simulink model "core1_simulator"  (R2024b)
settings: Solver=FixedStepDiscrete  StartTime=0.0  StopTime=50  FixedStep=0.001  RelTol=1e-3
undefined symbols (not defined in the file): DiscIntNeverNeededParam, task_table_data
settings Model: Creator=bianca  LastModifiedBy=bianca
settings OptimizationCC: BlockReduction=off

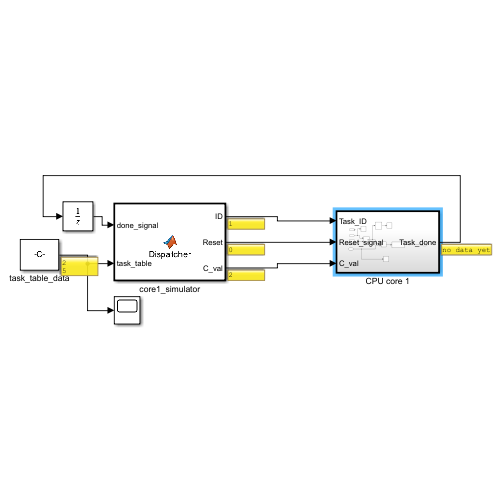
[thumbnail: Simulink's stored preview of the top-level diagram]
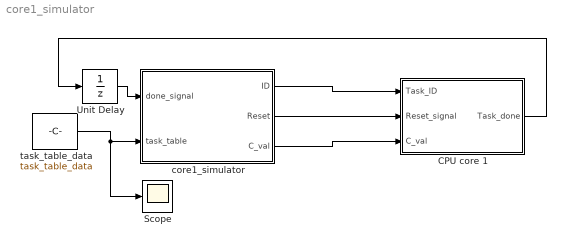
== system core1_simulator ==
  CPU core 1 : Subsystem  TreatAsAtomicUnit=on
  Scope : Scope
  Unit Delay : UnitDelay  SampleTime=0.001  HasFrameUpgradeWarning=on
  core1_simulator : MATLAB Function  TreatAsAtomicUnit=on
  task_table_data : Constant  Value=task_table_data  VectorParams1D=off  OutDataTypeStr=double  SampleTime=50
  wires:
  core1_simulator/1(ID) -> CPU core 1/1(Task_ID)
  core1_simulator/2(Reset) -> CPU core 1/2(Reset_signal)
  CPU core 1/1(Task_done) -> Unit Delay/1
  task_table_data/1 -> Scope/1, core1_simulator/2(task_table)
  Unit Delay/1 -> core1_simulator/1(done_signal)
  core1_simulator/3(C_val) -> CPU core 1/3(C_val)

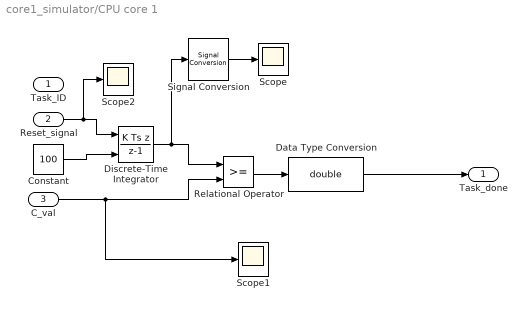
== system core1_simulator/CPU core 1 ==
  Task_ID : Inport
  Reset_signal : Inport  Port=2  PortDimensions=1
  C_val : Inport  Port=3  SampleTime=0.001
  Constant : Constant  Value=100  VectorParams1D=off  SampleTime=0.001
  Data Type Conversion : DataTypeConversion  OutDataTypeStr=double  SaturateOnIntegerOverflow=off  RndMeth=Floor
  Discrete-Time Integrator : DiscreteIntegrator  IntegratorMethod=Integration: Backward Euler  ExternalReset=rising  InitialCondition=0.001  SampleTime=0.001  ICPrevOutput=DiscIntNeverNeededParam  ICPrevScaledInput=DiscIntNeverNeededParam
  Relational Operator : RelationalOperator  OutDataTypeStr=boolean  RndMeth=Simplest  InputSameDT=off
  Scope : Scope
  Scope1 : Scope
  Scope2 : Scope
  Signal Conversion : SignalConversion  OverrideOpt=off
  Task_done : Outport
  wires:
  Reset_signal/1 -> Scope2/1, Discrete-Time Integrator/1
  Discrete-Time Integrator/1 -> Signal Conversion/1, Relational Operator/1
  Relational Operator/1 -> Data Type Conversion/1
  Data Type Conversion/1 -> Task_done/1
  Constant/1 -> Discrete-Time Integrator/2
  C_val/1 -> Relational Operator/2, Scope1/1
  Signal Conversion/1 -> Scope/1

== matlab function core1_simulator/core1_simulator ==
  data: done_signal input size=1; ID output; task_table input; Reset output size=1; C_val output size=1
function [ID, Reset, C_val] = Dispatcher(done_signal, task_table)

    ID = 1.0;
    C_val = 0.0;
    Reset = 0.0;

    persistent current_idx;
    persistent last_done_state;

    if isempty(current_idx)
        current_idx = 1;
        last_done_state = 0;
    end

    current_done = double(any(done_signal > 0.5));

    if isempty(last_done_state)
        Reset = 0.0;
    elseif (current_done == 1) && (last_done_state == 0)
        current_idx = current_idx + 1;
        Reset = 1.0;
    else
        Reset = 0.0;
    end
    
    % task is done, move to the next one
    if (current_done == 1) && (last_done_state == 0)
        current_idx = current_idx + 1;
        Reset = 1.0;
    else
        Reset = 0.0;
    end
   
    num_tasks = size(task_table, 1);

    if current_idx > num_tasks
        current_idx = 1;
    end

    last_done_state = current_done;
    
    ID = double(current_idx);

    if current_idx <= num_tasks
        C_val = double(task_table(uint32(current_idx), 1));
    else
        C_val = 0.0;
    end

    idx = uint32(current_idx);
    
    val = task_table(idx, 1);
    C_val = reshape(double(val), 1, 1); 
    ID = reshape(double(current_idx), 1, 1);
    Reset = reshape(double(Reset), 1, 1);
end
